simulink model "zuiyou_15"  (R2018b)
settings: Solver=VariableStepAuto  StartTime=0.0  StopTime=40  RelTol=1e-3
undefined symbols (not defined in the file or in its folder): AI1, AI2, AO1, Dev1
libraries: opclib x4
settings Model: Creator=erange  LastModifiedBy=erange

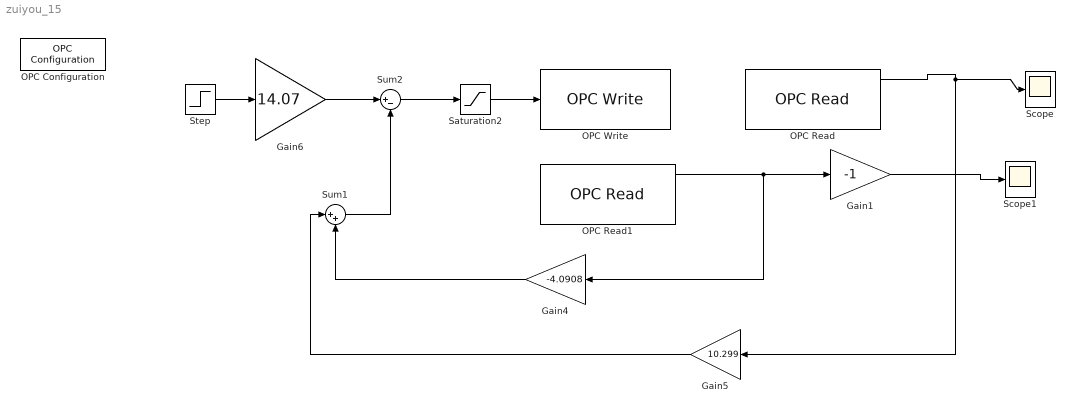
== system zuiyou_15 ==
  Gain1 : Gain  Gain=-1
  Gain4 : Gain  Gain=-4.0908
  Gain5 : Gain  Gain=10.299
  Gain6 : Gain  Gain=14.07
  OPC Configuration : opclib/OPC Configuration  opcServers=localhost/NI USB-6008.Server/10, localhost/Tank2.Server/10  errMissingItems=Error  errReadWrite=Warn  errShutdown=Error  errRTViolation=Warn  rtEnable=on  speedup=1  showLatency=off  beingUsed=on
      settings: SourceProductName=OPC Toolbox  SourceProductBaseCode=OT
  OPC Read : opclib/OPC Read  serverHost=localhost  serverID=NI USB-6008.Server  itemIDs=Dev1/AI1  readMode=Synchronous (cache)  dataType=double  updateRate=0.1  showQual=on  showTS=on  tsMode=Seconds since start
      settings: SourceProductName=OPC Toolbox  SourceProductBaseCode=OT
  OPC Read1 : opclib/OPC Read  serverHost=localhost  serverID=NI USB-6008.Server  itemIDs=Dev1/AI2  readMode=Synchronous (cache)  dataType=double  updateRate=0.1  showQual=on  showTS=on  tsMode=Seconds since start
      settings: SourceProductName=OPC Toolbox  SourceProductBaseCode=OT
  OPC Write : opclib/OPC Write  serverHost=localhost  serverID=NI USB-6008.Server  itemIDs=Dev1/AO1  writeMode=Synchronous  updateRate=0
      settings: SourceProductName=OPC Toolbox  SourceProductBaseCode=OT
  Saturation2 : Saturate  UpperLimit=5  LowerLimit=0
  Scope : Scope
  Scope1 : Scope
  Step : Step  Time=0  SampleTime=0
  Sum1 : Sum  Inputs=|++
  Sum2 : Sum  Inputs=|+-
  wires:
  Saturation2/1 -> OPC Write/1
  OPC Read/1 -> Gain5/1, Scope/1
  Step/1 -> Gain6/1
  Gain6/1 -> Sum2/1
  Sum2/1 -> Saturation2/1
  Sum1/1 -> Sum2/2
  OPC Read1/1 -> Gain1/1, Gain4/1
  Gain4/1 -> Sum1/2
  Gain5/1 -> Sum1/1
  Gain1/1 -> Scope1/1
